simulink model "fsr"  (Simulink 7.7)
settings: Solver=FixedStepDiscrete  StartTime=0.0  StopTime=inf  FixedStep=0.25  RelTol=1e-3
undefined symbols (not defined in the file): darwinop_communication_setup
libraries: simulink x2, lib_darwinop x1
settings Model: Creator=florent  LastModifiedBy=florent
settings DataIOCC: SignalLoggingSaveFormat=Dataset
settings OptimizationCC: ExpressionDepthLimit=128  OptimizeModelRefInitCode=on  LifeSpan=Inf
settings DebuggingCC: FcnCallInpInsideContextMsg=Enable All
settings HardwareCC: ProdEndianess=LittleEndian  ProdHWDeviceType=Generic->32-bit Embedded Processor
settings RTWCC: SystemTargetFile=darwinoplib.tlc  TemplateMakefile=darwinoplib.tmf  Description=DarwinOP code generator  ProcessScript=darwinoplib_make_rtw_hook  TargetLang=C++
settings CodeAppCC: IgnoreCustomStorageClasses=off  CustomSymbolStrType=$N$R$M_T
settings STFCustomTargetCC: TargetFunctionLibrary=C89/C90 (ANSI)  ERTCustomFileBanners=on  SupportContinuousTime=off  SupportNonInlinedSFcns=off  SystemTargetFile=darwinoplib.tlc
settings ERTTargetCC: TargetFunctionLibrary=C89/C90 (ANSI)  MultiwordLength=2048  ParMdlRefBuildCompliant=off  CompOptLevelCompliant=off  ERTFirstTimeCompliant=off  ModelStepFunctionPrototypeControlCompliant=off  CPPClassGenCompliant=off  InlinedParameterPlacement=NonHierarchical  ERTCustomFileTemplate=darwinoplib_main.tlc  ConvertIfToSwitch=off  SuppressUnreachableDefaultCases=off
settings CustomProperty: DataType=string  Value=192.168.123.1

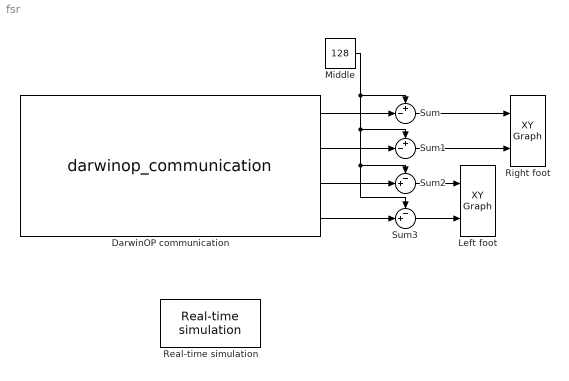
== system fsr ==
  DarwinOP communication : M-S-Function  StartFcn=darwinop_communication_setup('StartFcn');  StopFcn=darwinop_communication_setup('StopFcn');  FunctionName=darwinop_communication  Parameters=IP,Port,Protocol,Timeout,Frame,ReadIndex,WriteIndex  mask{IP=192.168.123.1, Port=1234, Protocol=tcp, Timeout=0.25, Frame=[ 2 111 34 2 2 112 34 2], ReadIndex=[ 1 1;2 1;3 1;4 1], WriteIndex=[]}
      settings: DeleteFcn=darwinop_communication_setup('DeleteFcn');  ModelCloseFcn=darwinop_communication_setup('ModelCloseFcn');  NameChangeFcn=darwinop_communication_setup('NameChangeFcn');  OpenFcn=darwinop_communication_setup('OpenFcn');
      mask StyleString: edit,edit,popup(tcp|udp),edit,edit,edit,edit
      mask Display:
      | image(imread('darwin-blk.jpg'))
      | 
      | port_label('output',1,'Pied droit(111)/Jauge X')
      | port_label('output',2,'Pied droit(111)/Jauge Y')
      | port_label('output',3,'Pied gauche(112)/Jauge X')
      | port_label('output',4,'Pied gauche(112)/Jauge Y')
  Left foot : simulink/Sinks/XY Graph  xmin=-128  xmax=128  ymin=-128  ymax=128  st=-1
  Middle : Constant  Value=128
  Real-time simulation : lib_darwinop/Real-time simulation  TimeScalingFactor=1
  Right foot : simulink/Sinks/XY Graph  xmin=-128  xmax=128  ymin=-128  ymax=128  st=-1
  Sum : Sum  Inputs=+-|
  Sum1 : Sum  Inputs=+-|
  Sum2 : Sum  Inputs=-+|
  Sum3 : Sum  Inputs=-+|
  wires:
  DarwinOP communication/1 -> Sum/2
  Sum/1 -> Right foot/1
  Sum1/1 -> Right foot/2
  DarwinOP communication/2 -> Sum1/2
  DarwinOP communication/3 -> Sum2/2
  DarwinOP communication/4 -> Sum3/2
  Sum2/1 -> Left foot/1
  Sum3/1 -> Left foot/2
  Middle/1 -> Sum/1, Sum1/1, Sum2/1, Sum3/1
